simulink model "dioderect"  (R2020b)
settings: Solver=VariableStepAuto  StartTime=0.0  StopTime=0.3  RelTol=1e-3
libraries: powerlib x13
settings Model: Creator=emin3  LastModifiedBy=emin3

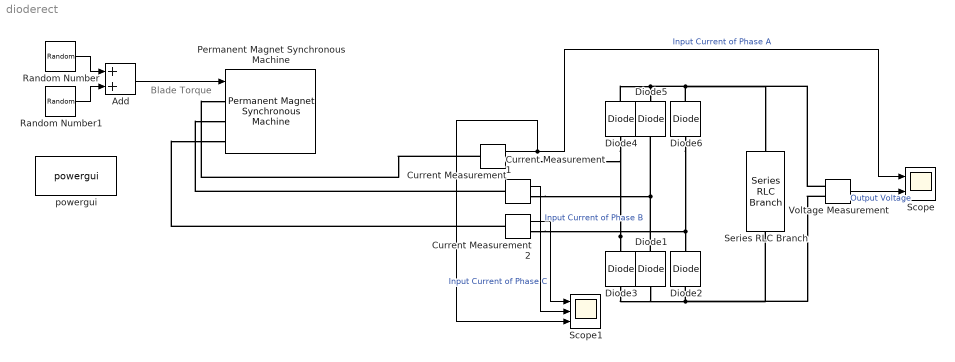
== system dioderect ==
  note: Blade Torque
  Add : Sum
  Current Measurement : powerlib/Measurements/Current Measurement  PhasorSimulation=off  OutputType=Complex  PSBequivalent=0
  Current Measurement1 : powerlib/Measurements/Current Measurement  PhasorSimulation=off  OutputType=Complex  PSBequivalent=0
  Current Measurement2 : powerlib/Measurements/Current Measurement  PhasorSimulation=off  OutputType=Complex  PSBequivalent=0
  Diode{1..6} (6 alike) : powerlib/Power Electronics/Diode  Ron=1e-9  Lon=0  Vf=0.8  IC=0  UseSnubber=0  Rs=1e-6  Cs=250e-9  Measurements=off
  Permanent Magnet Synchronous Machine : powerlib/Machines/Permanent Magnet Synchronous Machine  NbPhases=3  FluxDistribution=Sinusoidal  RotorType=Round  MechanicalLoad=Torque Tm  PresetModel=No  ShowDetailedParameters=on  MeasurementBus=off  Resistance=10.58  Inductance=8.5e-3  dqInductances=[8.5e-3,8.5e-3]  La=0.0167  MachineConstant=Voltage Constant (V_peak L-L / krpm)  Flux=0.60646  VoltageCst=110  TorqueCst=0.90969  Flat=120  Mechanical=[0.00027 0.005024 1 0]  PolePairs=4  InitialConditions=[300,0, 0,0]  InitialConditions5ph=[0 0 0 0 0 0]  RefAngle=90 degrees behind phase A axis (modified Park)  IterativeDiscreteModel=Trapezoidal non iterative  TsBlock=-1  TsPowergui=0
  Random Number : RandomNumber  Mean=-1.6  Variance=0.05  SampleTime=1
  Random Number1 : RandomNumber  Variance=0.1  SampleTime=1e-3
  Scope : Scope  NumInputPorts=2
  Scope1 : Scope  NumInputPorts=3
  Series RLC Branch : powerlib/Elements/Series RLC Branch  LConnTagsString=__new0  RConnTagsString=__new0  BranchType=R  Resistance=20  Inductance=1e-3  SetiL0=off  InitialCurrent=0  Capacitance=1e-6  Setx0=off  InitialVoltage=0  Measurements=None
  Voltage Measurement : powerlib/Measurements/Voltage Measurement  PhasorSimulation=off  OutputType=Complex  PSBequivalent=0
  powergui : powerlib/powergui  Priority=1  SimulationMode=Discrete  SampleTime=1e-7  frequency=60  Iterations=50  frequencyindice=0  Pbase=100e6  ErrMax=1e-4  UnitsV=kV  UnitsW=MW  buscounter=0  FunctionMessages=off  echomessages=off  EnableUseOfTLC=off  CurrentSourceSwitches=off  DisableSnubberDevices=off  DisableRonSwitches=off  DisableVfSwitches=off  DisplayEquations=off  AutomaticDiscreteSolvers=off  SolverType=Tustin/Backward Euler (TBE)  Interpol=off  ExternalGateDelay=off  methode=off  Ts=100  x0status=blocks  SPID=on  SwTol=0  HookPort=off  NonlinearTolerance=0  nMaxIteration=15  ContinueOnMaxIteration=off  RestoreLinks=warning  ResistiveCurrentMeasurement=off  Frange=[0:2:500]  Ylog=off  Xlog=on  ShowGrid=off  save=off  variable=ZData  structure=0  ZoomFFT=off  StartTime=0.0  cycles=1  DisplayStyle=1  fundamental=60  FreqAxis=off  MaxFrequency=1000  frequencyindicesteady=1  RmsSteady=1  display=off
  wires:
  Random Number/1 -> Add/1
  Add/1 -> Permanent Magnet Synchronous Machine/1
  Random Number1/1 -> Add/2
  Voltage Measurement/1 -> Scope/2  "Output Voltage"
  Current Measurement/1 -> Scope1/3, Scope/1  "Input Current of Phase A"
  Current Measurement2/1 -> Scope1/1  "Input Current of Phase C"
  Current Measurement1/1 -> Scope1/2  "Input Current of Phase B"
  connections:
  Diode6/LConn1 -- Current Measurement2/RConn1 -- Diode2/RConn1
  Diode2/LConn1 -- Voltage Measurement/LConn2 -- Series RLC Branch/RConn1 -- Diode3/LConn1 -- Diode1/LConn1
  Diode5/RConn1 -- Diode4/RConn1 -- Series RLC Branch/LConn1 -- Voltage Measurement/LConn1 -- Diode6/RConn1
  Diode1/RConn1 -- Current Measurement1/RConn1 -- Diode5/LConn1
  Diode3/RConn1 -- Diode4/LConn1 -- Current Measurement/RConn1
  Current Measurement/LConn1 -- Permanent Magnet Synchronous Machine/LConn1
  Current Measurement1/LConn1 -- Permanent Magnet Synchronous Machine/LConn2
  Current Measurement2/LConn1 -- Permanent Magnet Synchronous Machine/LConn3
